simulink model "FirstOrderEstim"  (R2021a)
settings: Solver=FixedStepAuto  StartTime=0.0  StopTime=tf  FixedStep=Ts  RelTol=1e-3
values from neighbouring files (symbols this model uses):
  a = 1    [Params.m]
  b = 2    [Params.m]
  den1 = [1 2*z*w w*w]    [Params.m]
  den2 = conv(den2,[tau 1])    [Params.m]
  num1 = [w*w]    [Params.m]
  num2 = [w*w]    [Params.m]
undefined symbols (not defined in the file or in its folder): Noise
libraries: simulink x1
settings Model: Creator=perruquetti  LastModifiedBy=perruquetti

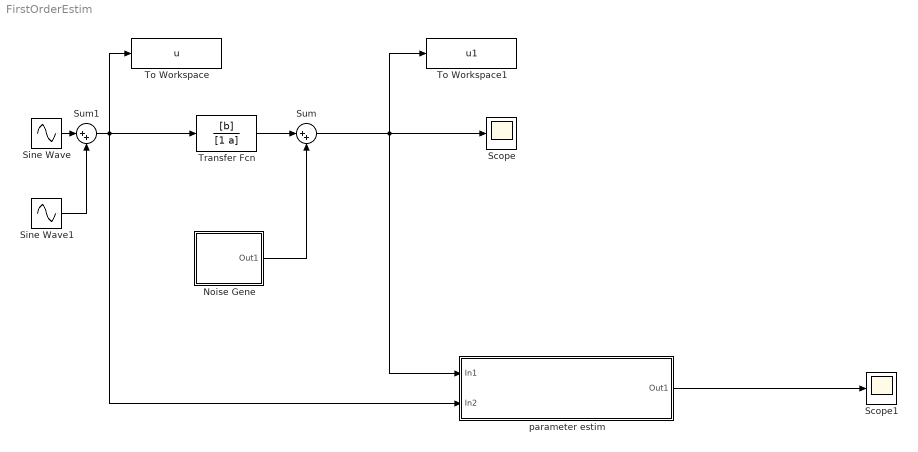
== system FirstOrderEstim ==
  Noise Gene : Subsystem
  Scope : Scope
  Scope1 : Scope
  Sine Wave : Sin  Amplitude=0.8  Frequency=10  SampleTime=0
  Sine Wave1 : Sin  Amplitude=0.8  Frequency=30  SampleTime=0
  Sum : Sum  Inputs=|++
  Sum1 : Sum  Inputs=|++
  To Workspace : ToWorkspace  VariableName=u  SampleTime=-1
  To Workspace1 : ToWorkspace  VariableName=u1  SampleTime=-1
  Transfer Fcn : TransferFcn  Numerator=[b]  Denominator=[1 a]
  parameter estim : Subsystem
  wires:
  Transfer Fcn/1 -> Sum/1
  Noise Gene/1(Out1) -> Sum/2
  Sum/1 -> parameter estim/1(In1), To Workspace1/1, Scope/1
  parameter estim/1(Out1) -> Scope1/1
  Sine Wave/1 -> Sum1/1
  Sum1/1 -> parameter estim/2(In2), To Workspace/1, Transfer Fcn/1
  Sine Wave1/1 -> Sum1/2

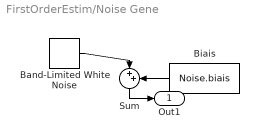
== system FirstOrderEstim/Noise Gene ==
  Band-Limited White Noise : simulink/Sources/Band-Limited White Noise  Cov=Noise.power  Ts=Noise.sampling  seed=Noise.seed
  Biais : Constant  Value=Noise.biais
  Sum : Sum  Inputs=|++
  Out1 : Outport
  wires:
  Sum/1 -> Out1/1
  Biais/1 -> Sum/2
  Band-Limited White Noise/1 -> Sum/1

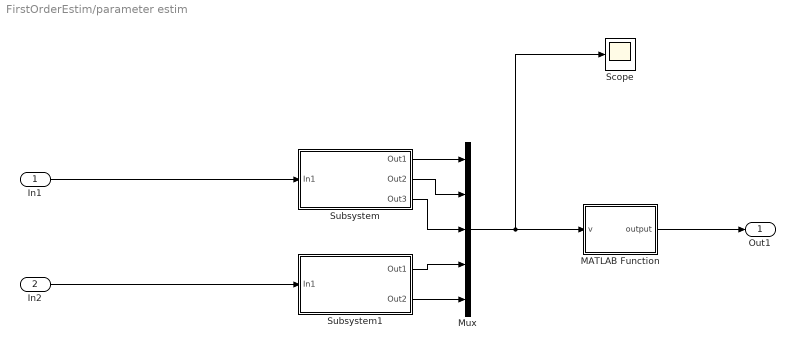
== system FirstOrderEstim/parameter estim ==
  In1 : Inport
  In2 : Inport  Port=2
  MATLAB Function : MATLAB Function  TreatAsAtomicUnit=on
  Mux : Mux  Inputs=5
  Scope : Scope
  Subsystem : Subsystem
  Subsystem1 : Subsystem
  Out1 : Outport
  wires:
  MATLAB Function/1(output) -> Out1/1
  Subsystem/3(Out3) -> Mux/3
  Subsystem/1(Out1) -> Mux/1
  Subsystem1/1(Out1) -> Mux/4
  Subsystem1/2(Out2) -> Mux/5
  Subsystem/2(Out2) -> Mux/2
  Mux/1 -> MATLAB Function/1(v), Scope/1
  In2/1 -> Subsystem1/1(In1)
  In1/1 -> Subsystem/1(In1)

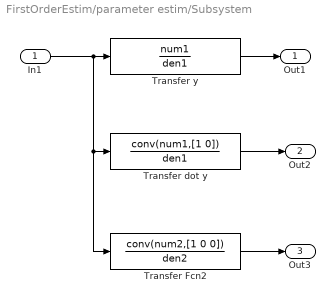
== system FirstOrderEstim/parameter estim/Subsystem ==
  In1 : Inport
  Transfer Fcn2 : TransferFcn  Numerator=conv(num2,[1 0 0])  Denominator=den2
  Transfer dot y : TransferFcn  Numerator=conv(num1,[1 0])  Denominator=den1
  Transfer y : TransferFcn  Numerator=num1  Denominator=den1
  Out1 : Outport
  Out2 : Outport  Port=2
  Out3 : Outport  Port=3
  wires:
  Transfer y/1 -> Out1/1
  In1/1 -> Transfer dot y/1, Transfer Fcn2/1, Transfer y/1
  Transfer Fcn2/1 -> Out3/1
  Transfer dot y/1 -> Out2/1

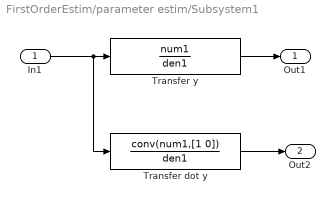
== system FirstOrderEstim/parameter estim/Subsystem1 ==
  In1 : Inport
  Transfer dot y : TransferFcn  Numerator=conv(num1,[1 0])  Denominator=den1
  Transfer y : TransferFcn  Numerator=num1  Denominator=den1
  Out1 : Outport
  Out2 : Outport  Port=2
  wires:
  Transfer y/1 -> Out1/1
  In1/1 -> Transfer dot y/1, Transfer y/1
  Transfer dot y/1 -> Out2/1

== matlab function FirstOrderEstim/parameter estim/MATLAB Function ==
  data: v input; output output
function output = fcn(v)
y=v(1);
doty=v(2);
ddoty=v(3);
u=v(4);
dotu=v(5);
A=[-y u;-doty dotu];
b=[doty;ddoty];

if isfinite(det(A)) & (abs(det(A))<100)
    y=pinv(A)*b;
else 
    y=[0;0];
end;
output = y;
